simulink model "ARO_UIO_alternative_2021_02_08"  (R2019b)
settings: Solver=FixedStepAuto  StartTime=0.0  StopTime=60  FixedStep=0.1  RelTol=1e-3
values from neighbouring files (symbols this model uses):
  Am = A_data{opt_order}    [ARO_UIO_balas_2021_02_08.m]
  B = B2    [ARO_UIO_balas_2021_02_08.m]
  C = C_data{opt_order}    [ARO_UIO_balas_2021_02_08.m]
  Fu = [0 0 0 0 0; 0 0 1 0 0;0 -25 0 0 0;0 0 0 0 1;0 0 0 -144 0]    [ARO_UIO_balas_2021_02_08.m]
  gamma_e = [0.0001;0.0001;0.0001;0.0001;0.0001;0.0001]'    [ARO_UIO_balas_2021_02_08.m]
  K_u = -rand(5,6)*randi([-10,-1])    [ARO_UIO_balas_2021_02_08.m]
  Theta = [1,1,1,1,1]    [ARO_UIO_balas_2021_02_08.m]
settings Model: Creator=Tris  LastModifiedBy=Tris
settings DataIOCC: ExternalInput="Y_sim1, Y_sim2, Y_sim3,  Y_sim4, Y_sim5, Y_sim6"  LoadExternalInput=on

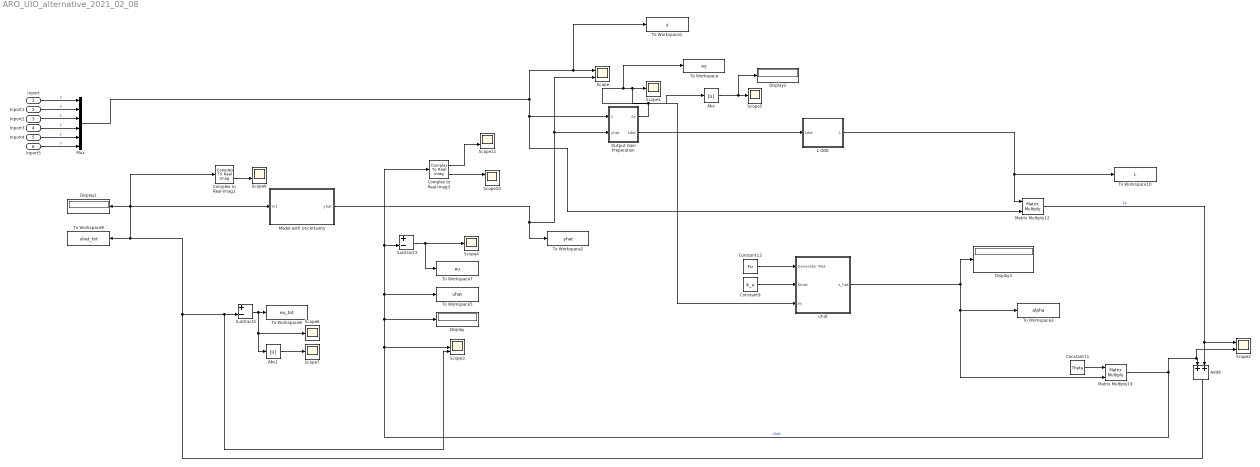
== system ARO_UIO_alternative_2021_02_08 ==
  Inport : Inport
  Inport1 : Inport  Port=2
  Inport2 : Inport  Port=3
  Inport3 : Inport  Port=4
  Inport4 : Inport  Port=5
  Inport5 : Inport  Port=6
  " L ODE" : Subsystem
  " uhat " : Subsystem
  Abs : Abs
  Abs1 : Abs
  Add6 : Sum
  Complex to Real-Imag1 : ComplexToRealImag
  Complex to Real-Imag3 : ComplexToRealImag
  Constant11 : Constant  Value=Theta  VectorParams1D=off
  Constant12 : Constant  Value=Fu
  Constant9 : Constant  Value=K_u  VectorParams1D=off
  Display{,1..3} (4 alike) : Display
  Matrix Multiply12 : Product  Multiplication=Matrix(*)
  Matrix Multiply19 : Product  Multiplication=Matrix(*)
  Model with Uncertainty : Subsystem
  Mux : Mux  Inputs=6
  Output Gain Preperation : Subsystem
  Scope{,2,9..11} (5 alike) : Scope  NumInputPorts=2
  Scope{1,4..7} (5 alike) : Scope
  Scope3 : Scope  NumInputPorts=3
  Subtract3 : Sum  Inputs=+-
  Subtract4 : Sum  Inputs=+-
  To Workspace : ToWorkspace  VariableName=ey  SaveFormat=Timeseries  SampleTime=-1
  To Workspace1 : ToWorkspace  VariableName=y  SaveFormat=Timeseries  SampleTime=-1
  To Workspace10 : ToWorkspace  VariableName=L  SaveFormat=Timeseries  SampleTime=-1
  To Workspace2 : ToWorkspace  VariableName=yhat  SaveFormat=Timeseries  SampleTime=-1
  To Workspace3 : ToWorkspace  VariableName=alpha  SaveFormat=Timeseries  SampleTime=-1
  To Workspace5 : ToWorkspace  VariableName=uhat  SaveFormat=Timeseries  SampleTime=-1
  To Workspace7 : ToWorkspace  VariableName=eu  SaveFormat=Timeseries  SampleTime=-1
  To Workspace8 : ToWorkspace  VariableName=eu_tot  SaveFormat=Timeseries  SampleTime=-1
  To Workspace9 : ToWorkspace  VariableName=uhat_tot  SaveFormat=Timeseries  SampleTime=-1
  wires:
  Constant11/1 -> Matrix Multiply19/1
  Matrix Multiply19/1 -> Scope2/2, Add6/1, To Workspace5/1, Complex to Real-Imag3/1, Subtract3/2, Display/1, Scope3/2  "uhat"
  Matrix Multiply12/1 -> Scope2/1, Add6/2  "Ly"
  Subtract4/1 -> Abs1/1, Scope6/1, To Workspace8/1
  Constant9/1 -> " uhat "/2(Kmat)
  Constant12/1 -> " uhat "/1(Generator Mat)
  " uhat "/1(z_hat) -> To Workspace3/1, Matrix Multiply19/2, Display3/1
  " L ODE"/1(L) -> To Workspace10/1, Matrix Multiply12/1
  Mux/1 -> Matrix Multiply12/2, Output Gain Preperation/1(y), To Workspace1/1, Scope/1
  Abs/1 -> Display2/1, Scope5/1
  Model with Uncertainty/1(yhat) -> To Workspace2/1, Scope/2, Output Gain Preperation/2(yhat)
  Add6/1 -> Complex to Real-Imag1/1, Model with Uncertainty/1(In1), Display1/1, To Workspace9/1, Scope3/3, Subtract4/2
  Subtract3/1 -> Scope4/1, To Workspace7/1
  Output Gain Preperation/1(ey) -> To Workspace/1, Abs/1, Scope1/1, " uhat "/3(ey)
  Output Gain Preperation/2(Ldot) -> " L ODE"/1(Ldot)
  Abs1/1 -> Scope7/1
  Complex to Real-Imag1/2 -> Scope9/2
  Complex to Real-Imag3/1 -> Scope11/2
  Complex to Real-Imag3/2 -> Scope10/1
  Inport/1 -> Mux/1  "y"
  Inport1/1 -> Mux/2  "y"
  Inport2/1 -> Mux/3  "y"
  Inport3/1 -> Mux/4  "y"
  Inport4/1 -> Mux/5  "y"
  Inport5/1 -> Mux/6  "y"

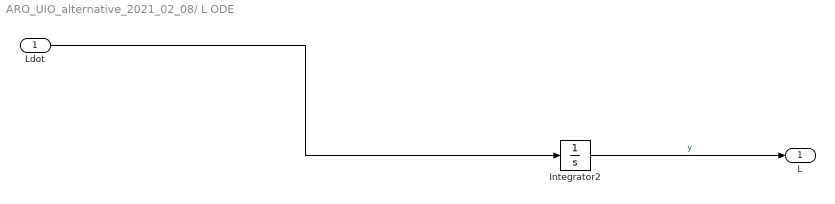
== system ARO_UIO_alternative_2021_02_08/ L ODE ==
  Ldot : Inport
  Integrator2 : Integrator
  L : Outport
  wires:
  Integrator2/1 -> L/1  "y"
  Ldot/1 -> Integrator2/1

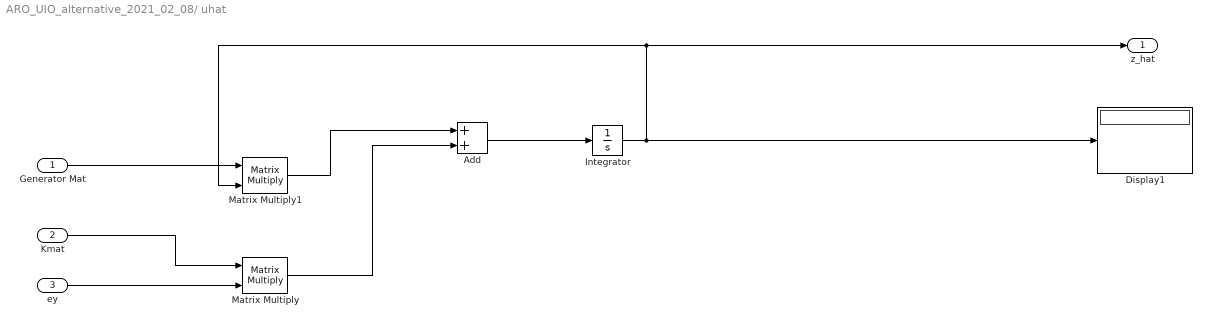
== system ARO_UIO_alternative_2021_02_08/ uhat  ==
  Generator Mat : Inport
  Kmat : Inport  Port=2
  ey : Inport  Port=3
  Add : Sum
  Display1 : Display
  Integrator : Integrator
  Matrix Multiply : Product  Multiplication=Matrix(*)
  Matrix Multiply1 : Product  Multiplication=Matrix(*)
  z_hat : Outport
  wires:
  ey/1 -> Matrix Multiply/2
  Kmat/1 -> Matrix Multiply/1
  Matrix Multiply/1 -> Add/2
  Add/1 -> Integrator/1
  Integrator/1 -> Display1/1, Matrix Multiply1/2, z_hat/1
  Generator Mat/1 -> Matrix Multiply1/1
  Matrix Multiply1/1 -> Add/1

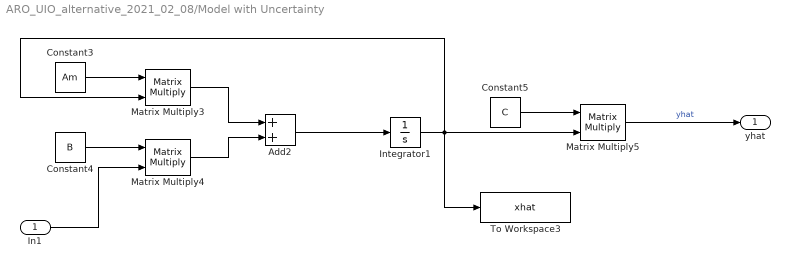
== system ARO_UIO_alternative_2021_02_08/Model with Uncertainty ==
  In1 : Inport
  Add2 : Sum
  Constant3 : Constant  Value=Am
  Constant4 : Constant  Value=B  VectorParams1D=off
  Constant5 : Constant  Value=C  VectorParams1D=off
  Integrator1 : Integrator
  Matrix Multiply3 : Product  Multiplication=Matrix(*)
  Matrix Multiply4 : Product  Multiplication=Matrix(*)
  Matrix Multiply5 : Product  Multiplication=Matrix(*)
  To Workspace3 : ToWorkspace  VariableName=xhat  SaveFormat=Timeseries  SampleTime=-1
  yhat : Outport
  wires:
  Constant3/1 -> Matrix Multiply3/1
  Integrator1/1 -> To Workspace3/1, Matrix Multiply5/2, Matrix Multiply3/2
  Constant5/1 -> Matrix Multiply5/1
  Add2/1 -> Integrator1/1
  Matrix Multiply4/1 -> Add2/2
  In1/1 -> Matrix Multiply4/2
  Constant4/1 -> Matrix Multiply4/1
  Matrix Multiply3/1 -> Add2/1
  Matrix Multiply5/1 -> yhat/1  "yhat"

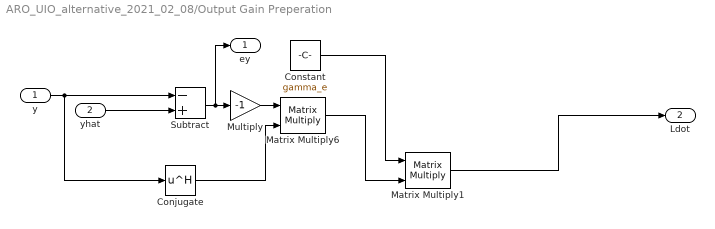
== system ARO_UIO_alternative_2021_02_08/Output Gain Preperation ==
  y : Inport
  yhat : Inport  Port=2
  Conjugate : Math  Operator=hermitian  RndMeth=Zero  SaturateOnIntegerOverflow=on
  Constant : Constant  Value=gamma_e  VectorParams1D=off
  Matrix Multiply1 : Product  Multiplication=Matrix(*)
  Matrix Multiply6 : Product  Multiplication=Matrix(*)
  Multiply : Gain  Gain=-1
  Subtract : Sum  Inputs=-+
  ey : Outport
  Ldot : Outport  Port=2
  wires:
  Matrix Multiply6/1 -> Matrix Multiply1/2
  Matrix Multiply1/1 -> Ldot/1
  Multiply/1 -> Matrix Multiply6/1
  Conjugate/1 -> Matrix Multiply6/2
  y/1 -> Conjugate/1, Subtract/1
  yhat/1 -> Subtract/2
  Subtract/1 -> Multiply/1, ey/1
  Constant/1 -> Matrix Multiply1/1
